simulink model "Black_box_system_2_1_1"  (R2024b)
settings: Solver=VariableStepAuto  StartTime=0.0  StopTime=45  FixedStep=0.001  RelTol=1e-3
undefined symbols (not defined in the file): degs2rpm, K_W, kd, ki, kp, rdp, rpm2degs, sens, simul, step_gain, tl, Ts, u_bar_max
libraries: simulink x2
settings Model: Creator=Enrico  LastModifiedBy=Enrico 2
settings DataIOCC: ReturnWorkspaceOutputsName=out_black_box

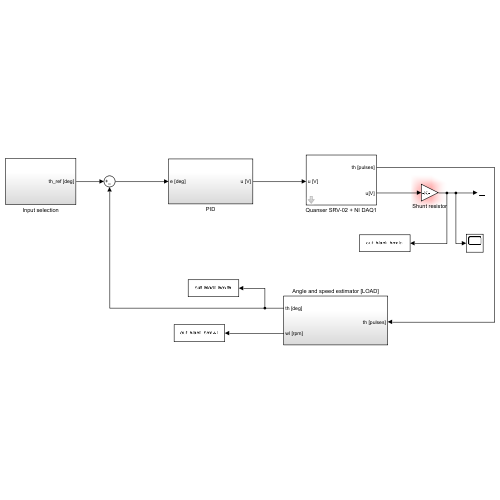
[thumbnail: Simulink's stored preview of the top-level diagram]
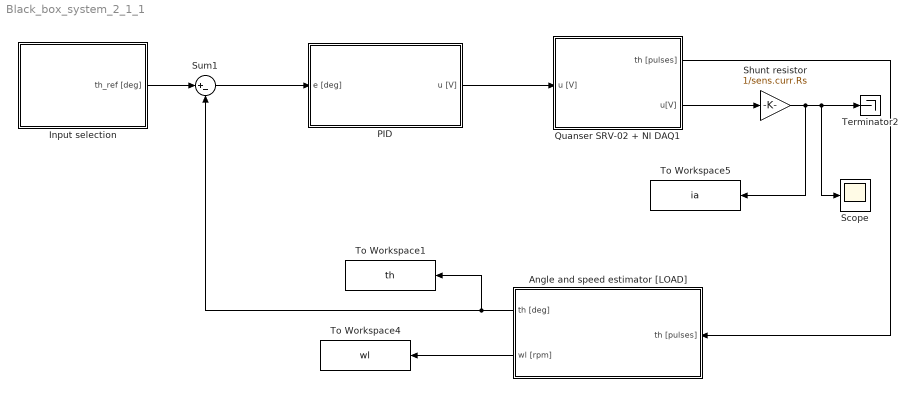
== system Black_box_system_2_1_1 ==
  Angle and speed estimator [LOAD] : Subsystem
  Input selection : Subsystem
  PID : Subsystem
  Quanser SRV-02 + NI DAQ1 : Subsystem  mask(Quanser SRV-02 (with inertial load) + NI DAQ){Ts=0.001, fricType=Karnopp}
      mask prompts: Ts "NI DAQ Sample Time:"; fricType "Friction model"
      mask help: Quanser SRV-02 (with inertial load) + NI DAQ model.
      mask init:
      | %%  Sensors data
      | 
      | %   shunt resistor
      | sens.curr.Rs = 0.5;                         %   resistance [Ohm]   
      | sens.curr.uRs_std = 0.01;                   %   voltage noise standard dev [V]                           
      | sens.curr.uRs_var = sens.curr.uRs_std^2;	%   voltage noise variance [V^2]
      | 
      | %   Hewlett-Packard HEDS-5540#A06 optical encoder
      | sens.enc.ppr = 500*4;                       %   pulses per rotation
      | sens.enc.pulse2deg = 360/sens.enc.ppr;      %   [pulses] -> [deg]
      | sens.enc.pulse2rad = 2*pi/sens.enc.ppr;     %   [pulses] -> [rad]
      | sens.enc.deg2pulse = sens.enc.ppr/360;      %   [deg] -> [pulses]
      | sens.enc.rad2pulse = sens.enc.ppr/2/pi;     %   [rad] -> [pulses]
      | 
      | 
      | %%  Data acquisition board (daq) data
      | 
      | %   NI PCI-6221 DAC data
      | daq.dac.bits = 16;                                  %   resolution (bits)
      | daq.dac.fs   = 10;                                  %   full scale 
      | daq.dac.q    = 2*daq.dac.fs/(2^daq.dac.bits-1);     %	quantization
      | 
      | %   NI PCI-6221 ADC data
      | daq.adc.bits = 16;                                  %   resolution (bits)
      | daq.adc.fs   = 10;                                  %   full scale (as set in SLDRT Analog Input block)
      | daq.adc.q    = 2*daq.adc.fs/(2^daq.adc.bits-1);     %   quantization
      mask Help:
      | Riccardo Antonello (antonello@dei.unipd.it)
      | 
      | April 24, 2020
      | 
      | Dept. of Information Engineering, University of Padova
      mask TypeOptions fricType: Coulomb + viscous | Karnopp
  Scope : Scope
  Shunt resistor : Gain  Gain=1/sens.curr.Rs
  Sum1 : Sum  Inputs=|+-
  Terminator2 : Terminator
  To Workspace1 : ToWorkspace  VariableName=th  SaveFormat=Structure With Time  SampleTime=0.001
  To Workspace4 : ToWorkspace  VariableName=wl  SaveFormat=Structure With Time  SampleTime=0.001
  To Workspace5 : ToWorkspace  VariableName=ia  SaveFormat=Structure With Time  SampleTime=0.001
  wires:
  Angle and speed estimator [LOAD]/1(th [deg]) -> To Workspace1/1, Sum1/2
  Quanser SRV-02 + NI DAQ1/2(u[V]) -> Shunt resistor/1
  Sum1/1 -> PID/1(e [deg])
  Angle and speed estimator [LOAD]/2(wl [rpm]) -> To Workspace4/1
  Quanser SRV-02 + NI DAQ1/1(th [pulses]) -> Angle and speed estimator [LOAD]/1(th [pulses])
  Shunt resistor/1 -> Scope/1, Terminator2/1, To Workspace5/1
  Input selection/1(th_ref [deg]) -> Sum1/1
  PID/1(u [V]) -> Quanser SRV-02 + NI DAQ1/1(u [V])

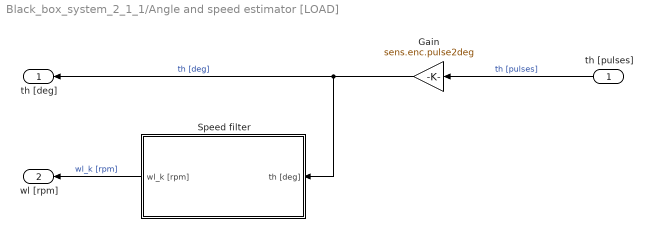
== system Black_box_system_2_1_1/Angle and speed estimator [LOAD] ==
  th [pulses] : Inport
  Gain : Gain  Gain=sens.enc.pulse2deg
  Speed filter : Subsystem
  th [deg] : Outport
  wl [rpm] : Outport  Port=2
  wires:
  Speed filter/1(wl_k [rpm]) -> wl [rpm]/1  "wl_k [rpm]"
  th [pulses]/1 -> Gain/1  "th [pulses]"
  Gain/1 -> Speed filter/1(th [deg]), th [deg]/1  "th [deg]"

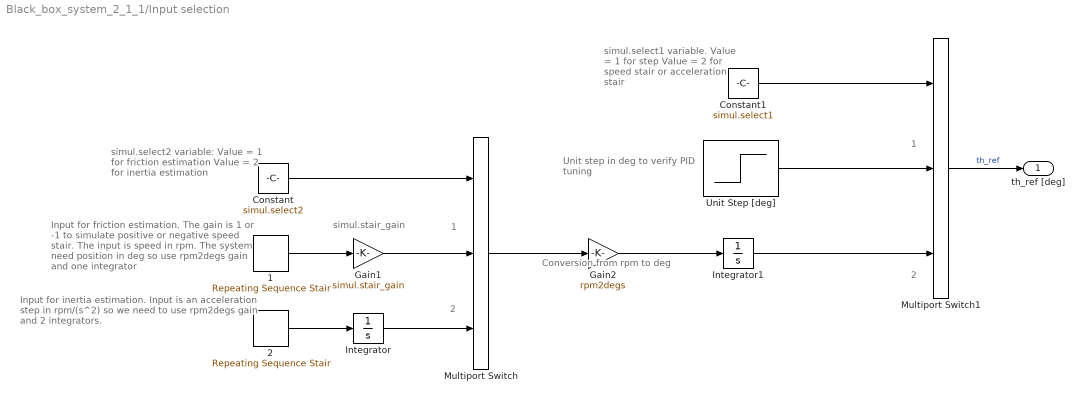
== system Black_box_system_2_1_1/Input selection ==
  note: Conversion from rpm to deg
  note: Input for friction estimation. The gain
      | is 1 or -1 to simulate positive or negative
      | speed stair. The input is speed in rpm.
      | The system need position in deg so use
      | rpm2degs gain and one integrator
  note: Input for inertia estimation. Input is an acceleration
      | step in rpm/(s^2) so we need to use
      | rpm2degs gain and 2 integrators.
  note: simul.select2 variable:
      | Value = 1 for friction estimation
      | Value = 2 for inertia estimation
  note: Unit step in deg to verify PID
      | tuning
  note: simul.select1 variable.
      | Value = 1 for step
      | Value = 2 for speed stair
      | or acceleration stair
  note: simul.stair_gain
  note: 1
  note: 2
  note: 1
  note: 2
  1 : simulink/Sources/Repeating Sequence Stair  OutValues=[50 100 150 200 250 300 350 400 450 450].'  tsamp=5  OutMin=[]  OutMax=[]  OutDataTypeStr=double  OutputDataTypeScalingMode=double  OutDataType=fixdt(0,8)  ConRadixGroup=Best Precision: Vector-wise  OutScaling=2^-12
  2 : simulink/Sources/Repeating Sequence Stair  OutValues=[450 -450].'  tsamp=1  OutMin=[]  OutMax=[]  OutDataTypeStr=double  OutputDataTypeScalingMode=double  OutDataType=fixdt(0,8)  ConRadixGroup=Best Precision: Vector-wise  OutScaling=2^-12
  Constant : Constant  Value=simul.select2
  Constant1 : Constant  Value=simul.select1
  Gain1 : Gain  Gain=simul.stair_gain
  Gain2 : Gain  Gain=rpm2degs
  Integrator : Integrator
  Integrator1 : Integrator
  Multiport Switch : MultiPortSwitch  Inputs=2  SaturateOnIntegerOverflow=off  InputSameDT=off
  Multiport Switch1 : MultiPortSwitch  Inputs=2  SaturateOnIntegerOverflow=off  InputSameDT=off
  Unit Step [deg] : Step  After=step_gain  SampleTime=Ts
  th_ref [deg] : Outport
  wires:
  Integrator1/1 -> Multiport Switch1/3
  Constant/1 -> Multiport Switch/1
  Gain1/1 -> Multiport Switch/2
  1/1 -> Gain1/1
  Gain2/1 -> Integrator1/1
  2/1 -> Integrator/1
  Unit Step [deg]/1 -> Multiport Switch1/2
  Constant1/1 -> Multiport Switch1/1
  Multiport Switch1/1 -> th_ref [deg]/1  "th_ref"
  Multiport Switch/1 -> Gain2/1
  Integrator/1 -> Multiport Switch/3

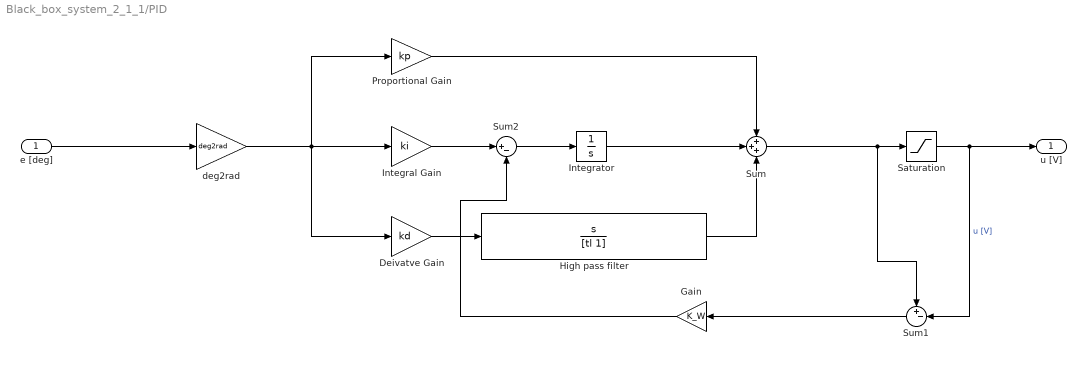
== system Black_box_system_2_1_1/PID ==
  e [deg] : Inport
  Deivatve Gain : Gain  Gain=kd
  Gain : Gain  Gain=K_W
  High pass filter : TransferFcn  Numerator=[1 0]  Denominator=[tl 1]
  Integral Gain : Gain  Gain=ki
  Integrator : Integrator
  Proportional Gain : Gain  Gain=kp
  "Saturation " : Saturate  UpperLimit=u_bar_max  LowerLimit=-u_bar_max
  Sum : Sum  Inputs=+++
  Sum1 : Sum  Inputs=+-|
  Sum2 : Sum  Inputs=|+-
  deg2rad : Gain  Gain=deg2rad
  u [V] : Outport
  wires:
  Deivatve Gain/1 -> High pass filter/1
  e [deg]/1 -> deg2rad/1
  Integrator/1 -> Sum/2
  "Saturation "/1 -> Sum1/2, u [V]/1  "u [V]"
  deg2rad/1 -> Deivatve Gain/1, Proportional Gain/1, Integral Gain/1
  High pass filter/1 -> Sum/3
  Proportional Gain/1 -> Sum/1
  Sum/1 -> Sum1/1, "Saturation "/1
  Sum1/1 -> Gain/1
  Integral Gain/1 -> Sum2/1
  Sum2/1 -> Integrator/1
  Gain/1 -> Sum2/2

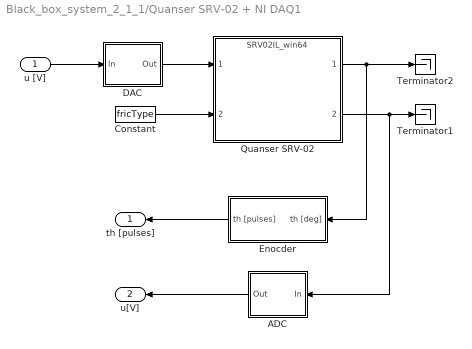
== system Black_box_system_2_1_1/Quanser SRV-02 + NI DAQ1 ==
  u [V] : Inport
  ADC : Subsystem
  Constant : Constant  Value=fricType
  DAC : Subsystem
  Enocder : Subsystem
  Quanser SRV-02 : ModelReference  ModelNameDialog=SRV02IL_win64.slxp  ModelReferenceVersion=1.44  CopyOfModelProtected=on
  Terminator1 : Terminator
  Terminator2 : Terminator
  th [pulses] : Outport
  u[V] : Outport  Port=2
  wires:
  Enocder/1(th [pulses]) -> th [pulses]/1
  ADC/1(Out) -> u[V]/1
  DAC/1(Out) -> Quanser SRV-02/1
  Quanser SRV-02/2 -> ADC/1(In), Terminator1/1
  u [V]/1 -> DAC/1(In)
  Quanser SRV-02/1 -> Enocder/1(th [deg]), Terminator2/1
  Constant/1 -> Quanser SRV-02/2

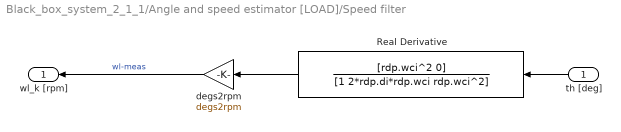
== system Black_box_system_2_1_1/Angle and speed estimator [LOAD]/Speed filter ==
  th [deg] : Inport
  Real Derivative : TransferFcn  Numerator=[rdp.wci^2 0]  Denominator=[1 2*rdp.di*rdp.wci rdp.wci^2]
  degs2rpm : Gain  Gain=degs2rpm
  wl_k [rpm] : Outport
  wires:
  th [deg]/1 -> Real Derivative/1
  degs2rpm/1 -> wl_k [rpm]/1  "wl-meas"
  Real Derivative/1 -> degs2rpm/1

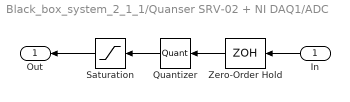
== system Black_box_system_2_1_1/Quanser SRV-02 + NI DAQ1/ADC ==
  In : Inport
  Quantizer : Quantizer  QuantizationInterval=daq.adc.q
  Saturation : Saturate  UpperLimit=daq.adc.fs  LowerLimit=-daq.adc.fs
  Zero-Order Hold : ZeroOrderHold  SampleTime=Ts
  Out : Outport
  wires:
  Saturation/1 -> Out/1
  In/1 -> Zero-Order Hold/1
  Quantizer/1 -> Saturation/1
  Zero-Order Hold/1 -> Quantizer/1

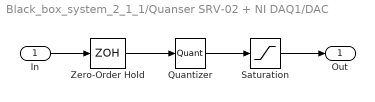
== system Black_box_system_2_1_1/Quanser SRV-02 + NI DAQ1/DAC ==
  In : Inport
  Quantizer : Quantizer  QuantizationInterval=daq.dac.q
  Saturation : Saturate  UpperLimit=daq.dac.fs  LowerLimit=-daq.dac.fs
  Zero-Order Hold : ZeroOrderHold  SampleTime=Ts
  Out : Outport
  wires:
  Quantizer/1 -> Saturation/1
  In/1 -> Zero-Order Hold/1
  Zero-Order Hold/1 -> Quantizer/1
  Saturation/1 -> Out/1

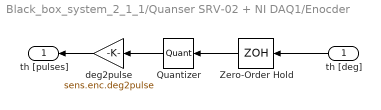
== system Black_box_system_2_1_1/Quanser SRV-02 + NI DAQ1/Enocder ==
  th [deg] : Inport
  Quantizer : Quantizer  QuantizationInterval=sens.enc.pulse2deg
  Zero-Order Hold : ZeroOrderHold  SampleTime=Ts
  deg2pulse : Gain  Gain=sens.enc.deg2pulse
  th [pulses] : Outport
  wires:
  Quantizer/1 -> deg2pulse/1
  th [deg]/1 -> Zero-Order Hold/1
  Zero-Order Hold/1 -> Quantizer/1
  deg2pulse/1 -> th [pulses]/1
